simulink model "PID_Joint23_Simscape_Simulation"  (R2020b)
settings: Solver=ode2  StartTime=0.0  StopTime=20  FixedStep=Ts  RelTol=1e-3
model workspace (MAT data in the model file):
  Ts = 0.001
undefined symbols (not defined in the file): DiscIntNeverNeededParam, PositionControl, TorqueControl, X, Y, Z
libraries: sm_lib x112, nesl_utility x65, simulink x4, dspsrcs4 x2
(part 1 of 4)
settings Model: Creator=Jeason  LastModifiedBy=Administrator
settings DataIOCC: InspectSignalLogs=on  ReturnWorkspaceOutputs=off
settings DebuggingCC: ArithmeticOperatorsInVariantConditions=warning
settings SFSimCC: CustomCodeUndefinedFunction=UseInterfaceOnly

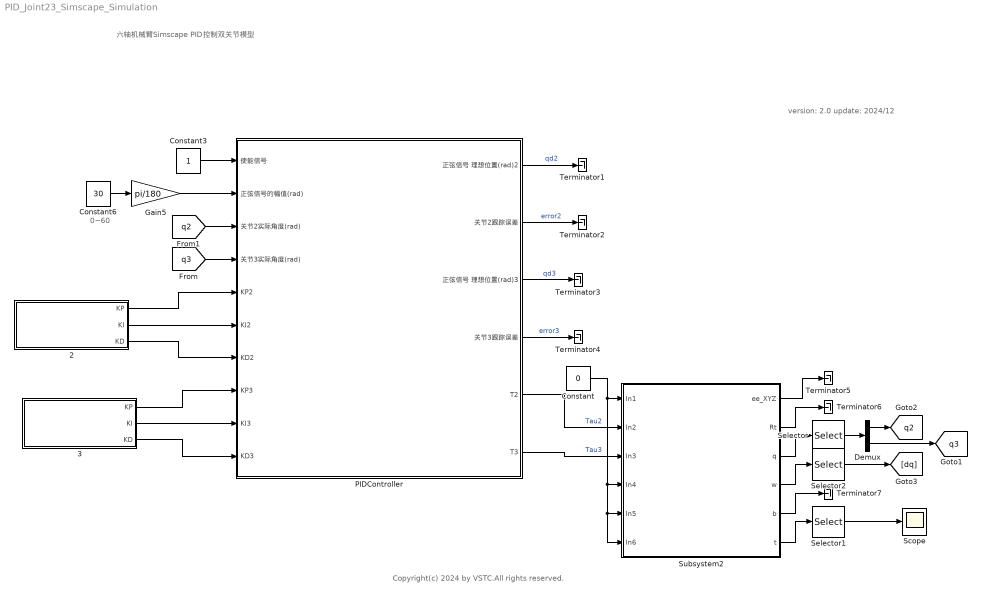
== system PID_Joint23_Simscape_Simulation ==
  note: 0~60
  note: 六轴机械臂Simscape PID控制双关节模型
  note: Copyright(c) 2024 by VSTC.All rights reserved.
  note: version: 2.0
      | update: 2024/12
  2 : Subsystem  mask{KP=300, KI=5, KD=10}
      mask DialogControl ParameterGroupVar Prompt: 参数
      mask Display: disp('PID parameters of Joint 2');
  3 : Subsystem  mask{KP=150, KI=5, KD=10}
      mask DialogControl ParameterGroupVar Prompt: 参数
      mask Display: disp('PID parameters of Joint 3');
  Constant : Constant  Value=0
  Constant3 : Constant
  Constant6 : Constant  Value=30
  Demux : Demux  Outputs=2
  Gain5 : Gain  Gain=pi/180
  PIDController : Subsystem  Priority=3  TreatAsAtomicUnit=on  RTWFcnName=AdaptiveAlgorithm
      settings: RTWSystemCode=Nonreusable function  RTWFcnNameOpts=User specified  RTWFileNameOpts=Use function name
  Scope : Scope
  Selector : Selector  InputPortWidth=6  IndexOptions=Index vector (dialog)  Indices=[2 3]  OutputSizes=1
  Selector1 : Selector  InputPortWidth=6  IndexOptions=Index vector (dialog)  Indices=3  OutputSizes=1
  Selector2 : Selector  InputPortWidth=6  IndexOptions=Index vector (dialog)  Indices=[2 3]  OutputSizes=1
  Subsystem2 : Subsystem  mask{VChoice1=PositionControl, VChoice2=TorqueControl, VChoice3=TorqueControl, VChoice4=PositionControl, VChoice5=PositionControl, VChoice6=PositionControl}
      mask prompts: VChoice1 "Select Joint1 Control Model"; VChoice2 "Select Joint2 Control Model"; VChoice3 "Select Joint3 Control Model"; VChoice4 "Select Joint4 Control Model"; VChoice5 "Select Joint5 Control Model"; VChoice6 "Select Joint6 Control Model"
      mask help: Model Choice
      mask TypeOptions VChoice1: Joint1/Variant Subsystem3/VChoice1
      mask TypeOptions VChoice2: Joint2/Variant Subsystem4/VChoice2
      mask TypeOptions VChoice3: Joint3/Variant Subsystem5/VChoice3
      mask TypeOptions VChoice4: Joint4/Variant Subsystem6/VChoice4
      mask TypeOptions VChoice5: Joint5/Variant Subsystem7/VChoice5
      mask TypeOptions VChoice6: Joint6/Variant Subsystem9/VChoice6
      mask Display:
      | % image('E:\SixRobotArm\Robot.png') ;
      | color('red');
      | disp('Six-DOF\n Collaborative Robot')
      | color('black');
      | choice1 = get_param(gcb,'VChoice1');
      | choice2 = get_param(gcb,'VChoice2');
      | choice3 = get_param(gcb,'VChoice3');
      | choice4 = get_param(gcb,'VChoice4');
      | choice5 = get_param(gcb,'VChoice5');
      | choice6 = get_param(gcb,'VChoice6');
      | if strcmp(choice1,'PositionControl') %TorqueControl
      |     port_label('input', 1, 'Theta1(rad)');
      | else
      |     port_label('input', 1, 'Torque1(N·m)');
      | end
      | if strcmp(choice2,'PositionControl') %TorqueControl
      |     port_label('input', 2, 'Theta2(rad)');
      | else
      |     port_label('input', 2, 'Torque2(N·m)');
      | end
      | if strcmp(choice3,'PositionControl') %TorqueControl
      |     port_label('input', 3, 'Theta3(rad)');
      | else
      |     port_label('input', 3, 'Torque3(N·m)');
      | end
      | if strcmp(choice4,'PositionControl') %TorqueControl
      |     port_label('input', 4, 'Theta4(rad)');
      | else
      |     port_label('input', 4, 'Torque4(N·m)');
      | end
      | if strcmp(choice5,'PositionControl') %TorqueControl
      |     port_label('input', 5, 'Theta5(rad)');
      | else
      |     port_label('input', 5, 'Torque5(N·m)');
      | end
      | if strcmp(choice6,'PositionControl') %TorqueControl
      |     port_label('input', 6, 'Theta6(rad)');
      | else
      |     port_label('input', 6, 'Torque6(N·m)');
      | end
      | 
      | port_label('output', 1, 'ee_XYZ(mm)');
      | port_label('output', 2, 'Rotation matrix');
      | port_label('output', 3, 'Angle(rad)');
      | port_label('output', 4, 'Vel(rad/s)');
      | port_label('output', 5, 'Acc(rad/s^2)');
      | port_label('output', 6, 'Torque(N·m)');
  Terminator{1..7} (7 alike) : Terminator
  tag scope: q2=global, q3=global
  wires:
  Gain5/1 -> PIDController/2(正弦信号的幅值(rad))
  Constant6/1 -> Gain5/1
  Constant3/1 -> PIDController/1(使能信号)
  [q3] -> PIDController/4(关节3实际角度(rad))
  [q2] -> PIDController/3(关节2实际角度(rad))
  2/1(KP) -> PIDController/5(KP2)
  2/2(KI) -> PIDController/6(KI2)
  2/3(KD) -> PIDController/7(KD2)
  3/1(KP) -> PIDController/8(KP3)
  3/2(KI) -> PIDController/9(KI3)
  3/3(KD) -> PIDController/10(KD3)
  PIDController/1(正弦信号 理想位置(rad)2) -> Terminator1/1  "qd2"
  PIDController/2(关节2跟踪误差) -> Terminator2/1  "error2"
  PIDController/3(正弦信号 理想位置(rad)3) -> Terminator3/1  "qd3"
  PIDController/4(关节3跟踪误差) -> Terminator4/1  "error3"
  Selector/1 -> Demux/1
  Selector1/1 -> Scope/1
  Selector2/1 -> [dq]
  Constant/1 -> Subsystem2/1(In1), Subsystem2/6(In6), Subsystem2/5(In5), Subsystem2/4(In4)
  Demux/1 -> [q2]
  Demux/2 -> [q3]
  Subsystem2/1(ee_XYZ) -> Terminator5/1
  Subsystem2/2(Rt) -> Terminator6/1
  Subsystem2/3(q) -> Selector/1
  Subsystem2/4(w) -> Selector2/1
  Subsystem2/5(b) -> Terminator7/1
  Subsystem2/6(t) -> Selector1/1
  PIDController/6(T3) -> Subsystem2/3(In3)  "Tau3"
  PIDController/5(T2) -> Subsystem2/2(In2)  "Tau2"

== system PID_Joint23_Simscape_Simulation/2 ==
  Constant : Constant  Value=KP
  Constant1 : Constant  Value=KI
  Constant2 : Constant  Value=KD
  KP : Outport
  KI : Outport  Port=2
  KD : Outport  Port=3
  wires:
  Constant/1 -> KP/1
  Constant1/1 -> KI/1
  Constant2/1 -> KD/1

== system PID_Joint23_Simscape_Simulation/3 ==
  Constant : Constant  Value=KP
  Constant1 : Constant  Value=KI
  Constant2 : Constant  Value=KD
  KP : Outport
  KI : Outport  Port=2
  KD : Outport  Port=3
  wires:
  Constant1/1 -> KI/1
  Constant2/1 -> KD/1
  Constant/1 -> KP/1

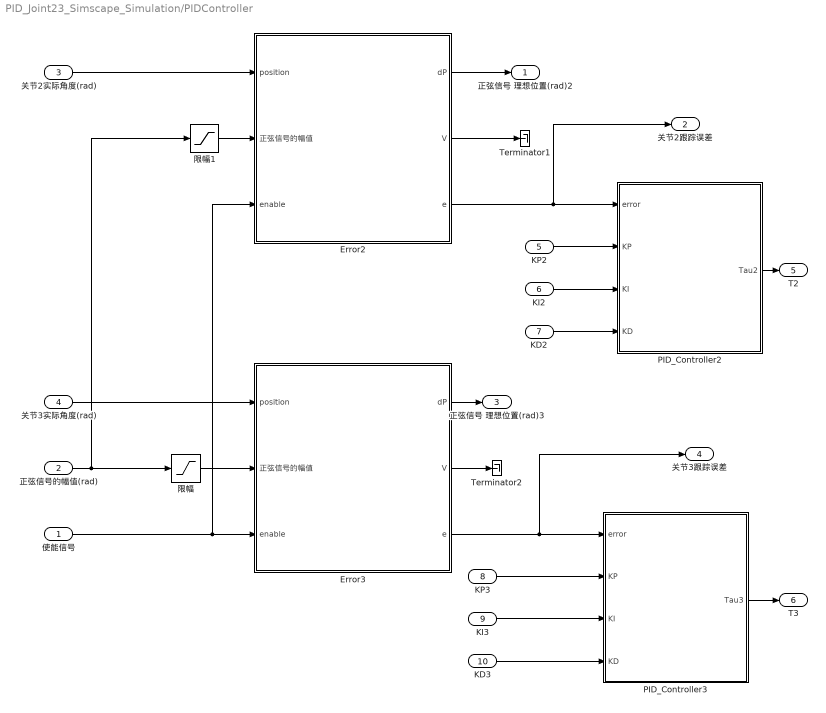
== system PID_Joint23_Simscape_Simulation/PIDController ==
  使能信号 : Inport
  正弦信号的幅值(rad) : Inport  Port=2
  关节2实际角度(rad) : Inport  Port=3
  关节3实际角度(rad) : Inport  Port=4
  KP2 : Inport  Port=5
  KI2 : Inport  Port=6
  KD2 : Inport  Port=7
  KP3 : Inport  Port=8
  KI3 : Inport  Port=9
  KD3 : Inport  Port=10
  Error2 : Subsystem  Priority=1  TreatAsAtomicUnit=on
      settings: RTWSystemCode=Nonreusable function  RTWFcnNameOpts=Use subsystem name  FunctionInterfaceSpec=Allow arguments (Optimized)
  Error3 : Subsystem  Priority=1  TreatAsAtomicUnit=on
      settings: RTWSystemCode=Nonreusable function  RTWFcnNameOpts=Use subsystem name  FunctionInterfaceSpec=Allow arguments (Optimized)
  PID_Controller2 : Subsystem  TreatAsAtomicUnit=on
      settings: RTWSystemCode=Nonreusable function
  PID_Controller3 : Subsystem  TreatAsAtomicUnit=on
      settings: RTWSystemCode=Nonreusable function
  Terminator1 : Terminator
  Terminator2 : Terminator
  限幅 : Saturate  UpperLimit=pi/3  LowerLimit=0
  限幅1 : Saturate  UpperLimit=pi/3  LowerLimit=0
  正弦信号 理想位置(rad)2 : Outport  VectorParamsAs1DForOutWhenUnconnected=off
  关节2跟踪误差 : Outport  Port=2  VectorParamsAs1DForOutWhenUnconnected=off
  正弦信号 理想位置(rad)3 : Outport  Port=3  VectorParamsAs1DForOutWhenUnconnected=off
  关节3跟踪误差 : Outport  Port=4  VectorParamsAs1DForOutWhenUnconnected=off
  T2 : Outport  Port=5  VectorParamsAs1DForOutWhenUnconnected=off
  T3 : Outport  Port=6  VectorParamsAs1DForOutWhenUnconnected=off
  wires:
  关节3实际角度(rad)/1 -> Error3/1(position)
  限幅/1 -> Error3/2(正弦信号的幅值)
  使能信号/1 -> Error2/3(enable), Error3/3(enable)
  Error3/3(e) -> 关节3跟踪误差/1, PID_Controller3/1(error)
  KP3/1 -> PID_Controller3/2(KP)
  KI3/1 -> PID_Controller3/3(KI)
  KD3/1 -> PID_Controller3/4(KD)
  Error3/1(dP) -> 正弦信号 理想位置(rad)3/1
  Error3/2(V) -> Terminator2/1
  Error2/3(e) -> 关节2跟踪误差/1, PID_Controller2/1(error)
  Error2/1(dP) -> 正弦信号 理想位置(rad)2/1
  Error2/2(V) -> Terminator1/1
  关节2实际角度(rad)/1 -> Error2/1(position)
  限幅1/1 -> Error2/2(正弦信号的幅值)
  KD2/1 -> PID_Controller2/4(KD)
  KI2/1 -> PID_Controller2/3(KI)
  KP2/1 -> PID_Controller2/2(KP)
  PID_Controller3/1(Tau3) -> T3/1
  PID_Controller2/1(Tau2) -> T2/1
  正弦信号的幅值(rad)/1 -> 限幅/1, 限幅1/1

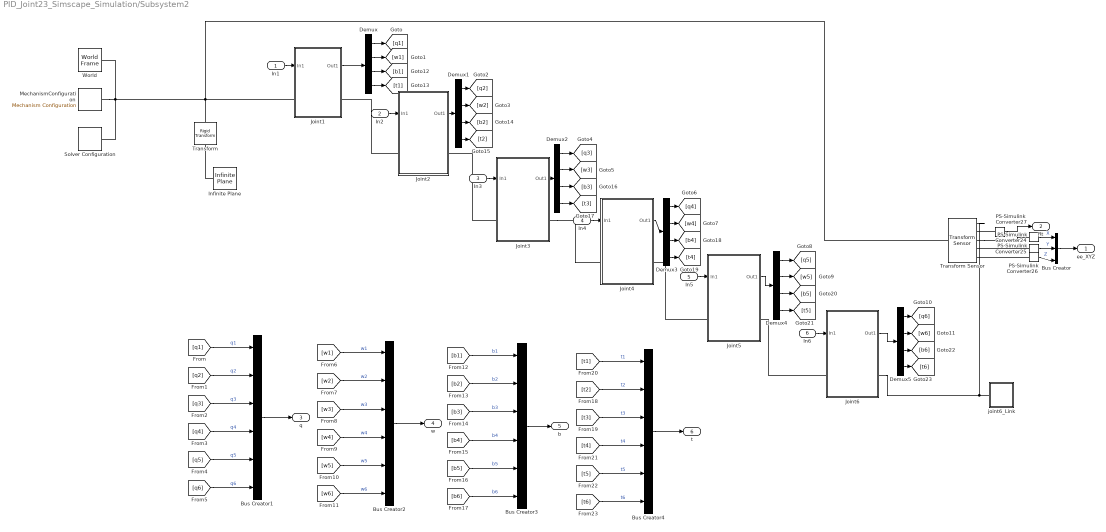
== system PID_Joint23_Simscape_Simulation/Subsystem2 ==
  In1 : Inport
  In2 : Inport  Port=2
  In3 : Inport  Port=3
  In4 : Inport  Port=4
  In5 : Inport  Port=5
  In6 : Inport  Port=6
  Bus Creator : BusCreator  Inputs=3
  Bus Creator{1..4} (4 alike) : BusCreator  Inputs=6
  Demux{,1..5} (6 alike) : Demux
  Infinite Plane : sm_lib/Curves and Surfaces/Infinite Plane  GraphicType=Rectangle  GraphicPlaneWidth=1  GraphicPlaneWidthUnits=m  GraphicPlaneHeight=1  GraphicPlaneHeightUnits=m  GraphicVisPropType=SimpleVisualProperties  GraphicDiffuseColor=[0.5 0.5 0.5]  GraphicOpacity=1  GraphicSpecularColor=[0.5 0.5 0.5 1.0]  GraphicAmbientColor=[0.15 0.15 0.15 1.0]  GraphicEmissiveColor=[0.0 0.0 0.0 1.0]  GraphicShininess=75
  Joint1 : Subsystem
  Joint2 : Subsystem
  Joint3 : Subsystem
  Joint4 : Subsystem
  Joint5 : Subsystem
  Joint6 : Subsystem
  MechanismConfiguration : sm_lib/Utilities/Mechanism Configuration  UniformGravity=Constant  GravityVector=[0 0 -9.80665]  GravityVectorUnits=m/s^2  GravityUnits=m/s^2  LinearizationDelta=0.001  JointModeTransitionNonlinearIterations=2
  PS-Simulink Converter{24..27} (4 alike) : nesl_utility/PS-Simulink Converter  PhysicalDomain=network_engine_domain  SubClassName=ps_output  LeftPortType=input  RightPortType=output  PseudoPeriodic=off  Frequencies=[]  Unit=mm  AffineConversion=off
      settings: SourceProductBaseCode=PW,SS
  Solver Configuration : nesl_utility/Solver Configuration  PhysicalDomain=network_engine_domain  SubClassName=solver  LeftPortType=input  RightPortType=generic  Tones=[]  Harmonics=[]  SimulateNoise=off  Profile=off  UseLocalSampling=off  EnableSwitchedLinearOptims=on  FrequencyDomain=off  UseCCode=off  RelTol=0.001  AbsTol=1e-06  MinStep=1e-09  ToWorkspace=off  RevertToSquareIcSolve=off  NumHomotopyIterations=100  PhasorMode=off  PhasorModeNumHarmonics=1  DoDC=off  ResidualTolerance=1e-09  UseLocalSolver=off  LocalSolverChoice=NE_BACKWARD_EULER_ADVANCER  LocalSolverSampleTime=0.001  DoFixedCost=off  MaxNonlinIter=3  MaxModeIter=2  ComputeImpulses=off  ImpulseIterations=2  LinearAlgebra=auto  EquationFormulation=NE_TIME_EF  DelaysMemoryBudget=1024  AutomaticFiltering=on  FilteringTimeConstant=0.001  PartitionStorageMethod=AS_NEEDED  PartitionMemoryBudget=1024  PartitionMethod=ROBUST
  Transform : sm_lib/Frames and Transforms/Rigid Transform  TranslationMethod=Cartesian  TranslationStandardOffset=0  TranslationLengthUnit=m  TranslationStandardAxis=+Z  TranslationCartesianOffset=[0, 0, 0]  TranslationROffset=0  TranslationROffsetUnits=m  TranslationZOffset=0  TranslationZOffsetUnits=m  TranslationThetaOffset=0  TranslationThetaOffsetUnits=deg  RotationMethod=RotationSequence  RotationAngleUnits=deg  RotationStandardAxis=+Z  RotationAngle=0.0  RotationArbitraryAxis=[0 0 1]  FollAlignAxisA=+X  BaseAlignAxisA=+Y  FollAlignAxisB=+Y  BaseAlignAxisB=+Z  RotationSequenceAxes=BaseAxes  RotationSequence=XYZ  RotationSequenceAngles=[0, 0, 0]  RotationSequenceAnglesUnits=rad  RotationMatrix=[1 0 0; 0 1 0; 0 0 1]
  Transform Sensor : sm_lib/Frames and Transforms/Transform Sensor  MeasurementFrame=Base  SenseAngle=off  SenseAxis=off  SenseAngle1=off  SenseAngle2=off  SenseAngle3=off  SenseQ=off  SenseR=on  SenseOmegaX=off  SenseOmegaY=off  SenseOmegaZ=off  SenseOmega1=off  SenseOmega2=off  SenseOmega3=off  SenseQDot=off  SenseRDot=off  SenseAlphaX=off  SenseAlphaY=off  SenseAlphaZ=off  SenseAlpha1=off  SenseAlpha2=off  SenseAlpha3=off  SenseQDDot=off  SenseRDDot=off  SenseX=on  SenseY=on  SenseZ=on  SenseRad=off  SenseAzim=off  SenseDist=off  SenseInc=off  SenseXDot=off  SenseYDot=off  SenseZDot=off  SenseRadDot=off  SenseAzimDot=off  SenseDistDot=off  SenseIncDot=off  SenseXDDot=off  SenseYDDot=off  SenseZDDot=off  SenseRadDDot=off  SenseAzimDDot=off  SenseDistDDot=off  SenseIncDDot=off
  World : sm_lib/Frames and Transforms/World Frame
  joint6_Link : Subsystem
  ee_XYZ : Outport
  Rt : Outport  Port=2
  q : Outport  Port=3
  w : Outport  Port=4
  b : Outport  Port=5
  t : Outport  Port=6
  wires:
  Demux4/4 -> [t5]
  PS-Simulink Converter25/1 -> Bus Creator/2  "Y"
  Joint3/1(Out1) -> Demux2/1
  Joint6/1(Out1) -> Demux5/1
  Demux3/4 -> [t4]
  PS-Simulink Converter26/1 -> Bus Creator/3  "Z"
  [q6] -> Bus Creator1/6  "q6"
  [b1] -> Bus Creator3/1  "b1"
  Joint4/1(Out1) -> Demux3/1
  [q1] -> Bus Creator1/1  "q1"
  Demux/3 -> [b1]
  Demux4/3 -> [b5]
  [t2] -> Bus Creator4/2  "t2"
  Bus Creator2/1 -> w/1
  Demux1/4 -> [t2]
  Joint1/1(Out1) -> Demux/1
  [w4] -> Bus Creator2/4  "w4"
  Demux4/2 -> [w5]
  Demux2/4 -> [t3]
  [q3] -> Bus Creator1/3  "q3"
  Demux/1 -> [q1]
  Demux1/3 -> [b2]
  [b5] -> Bus Creator3/5  "b5"
  Demux2/3 -> [b3]
  Demux2/1 -> [q3]
  [w3] -> Bus Creator2/3  "w3"
  [b2] -> Bus Creator3/2  "b2"
  [t5] -> Bus Creator4/5  "t5"
  [q4] -> Bus Creator1/4  "q4"
  Demux/2 -> [w1]
  Demux3/3 -> [b4]
  Bus Creator/1 -> ee_XYZ/1
  Demux5/3 -> [b6]
  [t6] -> Bus Creator4/6  "t6"
  Demux/4 -> [t1]
  Bus Creator1/1 -> q/1
  Demux5/1 -> [q6]
  [w6] -> Bus Creator2/6  "w6"
  PS-Simulink Converter27/1 -> Rt/1
  [w5] -> Bus Creator2/5  "w5"
  [q2] -> Bus Creator1/2  "q2"
  In4/1 -> Joint4/1(In1)
  In6/1 -> Joint6/1(In1)
  In5/1 -> Joint5/1(In1)
  [b3] -> Bus Creator3/3  "b3"
  Demux1/1 -> [q2]
  Demux3/1 -> [q4]
  In3/1 -> Joint3/1(In1)
  [q5] -> Bus Creator1/5  "q5"
  [w1] -> Bus Creator2/1  "w1"
  Bus Creator3/1 -> b/1
  PS-Simulink Converter24/1 -> Bus Creator/1  "X"
  [b6] -> Bus Creator3/6  "b6"
  [t3] -> Bus Creator4/3  "t3"
  [t1] -> Bus Creator4/1  "t1"
  [w2] -> Bus Creator2/2  "w2"
  Joint5/1(Out1) -> Demux4/1
  [t4] -> Bus Creator4/4  "t4"
  Demux1/2 -> [w2]
  Demux4/1 -> [q5]
  Demux2/2 -> [w3]
  In2/1 -> Joint2/1(In1)
  In1/1 -> Joint1/1(In1)
  Demux3/2 -> [w4]
  Joint2/1(Out1) -> Demux1/1
  Bus Creator4/1 -> t/1
  Demux5/2 -> [w6]
  [b4] -> Bus Creator3/4  "b4"
  Demux5/4 -> [t6]
  connections:
  Joint1/LConn1 -- World/RConn1 -- MechanismConfiguration/RConn1 -- Solver Configuration/RConn1 -- Transform/LConn1 -- Transform Sensor/LConn1
  Infinite Plane/LConn1 -- Transform/RConn1
  Transform Sensor/RConn3 -- PS-Simulink Converter24/LConn1
  PS-Simulink Converter27/LConn1 -- Transform Sensor/RConn2
  Joint3/RConn1 -- Joint4/LConn1
  Joint6/LConn1 -- Joint5/RConn1
  PS-Simulink Converter26/LConn1 -- Transform Sensor/RConn5
  PS-Simulink Converter25/LConn1 -- Transform Sensor/RConn4
  Joint2/LConn1 -- Joint1/RConn1
  Joint5/LConn1 -- Joint4/RConn1
  Joint3/LConn1 -- Joint2/RConn1
  Joint6/RConn1 -- Transform Sensor/RConn1 -- joint6_Link/LConn1

== system PID_Joint23_Simscape_Simulation/PIDController/Error2 ==
  note: $e_1(t)=\theta(t)-\theta_d(t)$
  note: $\dot\theta_d(t)$
  position : Inport
  正弦信号的幅值 : Inport  Port=2
  enable : Inport  Port=3
  Discrete Derivative : simulink/Discrete/Discrete Derivative  gainval=1.0  ICPrevScaledInput=0.0  OutMin=[]  OutMax=[]  OutDataType=fixdt(1, 16)  OutScaling=2^-10  DoSatur=off
  Subsystem : Subsystem
      settings: RTWSystemCode=Nonreusable function
  dP : Outport  VectorParamsAs1DForOutWhenUnconnected=off
  V : Outport  Port=2  VectorParamsAs1DForOutWhenUnconnected=off
  e : Outport  Port=3  VectorParamsAs1DForOutWhenUnconnected=off
  wires:
  position/1 -> Subsystem/1(position)
  Discrete Derivative/1 -> V/1
  enable/1 -> Subsystem/Enable
  Subsystem/2(理想位置) -> dP/1, Discrete Derivative/1
  Subsystem/1(e1) -> e/1
  正弦信号的幅值/1 -> Subsystem/2(Amplitude)

== system PID_Joint23_Simscape_Simulation/PIDController/Error3 ==
  note: $e_1(t)=\theta(t)-\theta_d(t)$
  note: $\dot\theta_d(t)$
  position : Inport
  正弦信号的幅值 : Inport  Port=2
  enable : Inport  Port=3
  Discrete Derivative : simulink/Discrete/Discrete Derivative  gainval=1.0  ICPrevScaledInput=0.0  OutMin=[]  OutMax=[]  OutDataType=fixdt(1, 16)  OutScaling=2^-10  DoSatur=off
  Subsystem : Subsystem
      settings: RTWSystemCode=Nonreusable function
  dP : Outport  VectorParamsAs1DForOutWhenUnconnected=off
  V : Outport  Port=2  VectorParamsAs1DForOutWhenUnconnected=off
  e : Outport  Port=3  VectorParamsAs1DForOutWhenUnconnected=off
  wires:
  position/1 -> Subsystem/1(position)
  Discrete Derivative/1 -> V/1
  enable/1 -> Subsystem/Enable
  Subsystem/2(理想位置) -> dP/1, Discrete Derivative/1
  Subsystem/1(e1) -> e/1
  正弦信号的幅值/1 -> Subsystem/2(Amplitude)

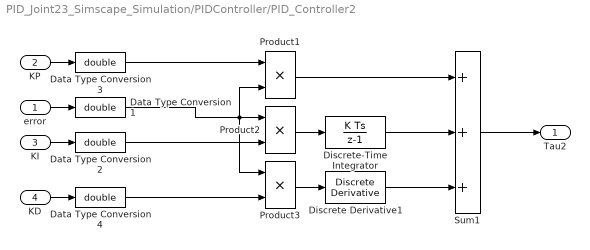
== system PID_Joint23_Simscape_Simulation/PIDController/PID_Controller2 ==
  error : Inport
  KP : Inport  Port=2
  KI : Inport  Port=3
  KD : Inport  Port=4
  Data Type Conversion{1..4} (4 alike) : DataTypeConversion  OutDataTypeStr=double
  Discrete Derivative1 : simulink/Discrete/Discrete Derivative  gainval=1.0  ICPrevScaledInput=0.0  OutMin=[]  OutMax=[]  OutDataType=fixdt(1, 16)  OutScaling=2^-10  DoSatur=off
  Discrete-Time Integrator : DiscreteIntegrator  SampleTime=-1  ICPrevOutput=DiscIntNeverNeededParam  ICPrevScaledInput=DiscIntNeverNeededParam
  Product1 : Product
  Product2 : Product
  Product3 : Product
  Sum1 : Sum  Inputs=+++
  Tau2 : Outport  VectorParamsAs1DForOutWhenUnconnected=off
  wires:
  Product2/1 -> Discrete-Time Integrator/1
  error/1 -> Data Type Conversion1/1
  Product3/1 -> Discrete Derivative1/1
  KP/1 -> Data Type Conversion3/1
  Sum1/1 -> Tau2/1
  Discrete Derivative1/1 -> Sum1/3
  Product1/1 -> Sum1/1
  Discrete-Time Integrator/1 -> Sum1/2
  KI/1 -> Data Type Conversion2/1
  KD/1 -> Data Type Conversion4/1
  Data Type Conversion3/1 -> Product1/1
  Data Type Conversion4/1 -> Product3/2
  Data Type Conversion2/1 -> Product2/2
  Data Type Conversion1/1 -> Product3/1, Product1/2, Product2/1

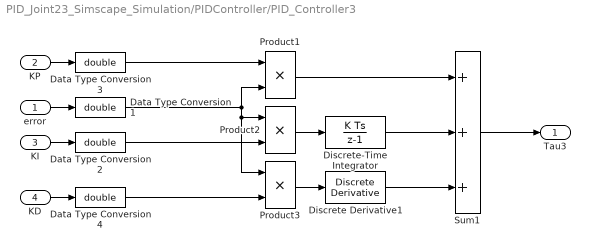
== system PID_Joint23_Simscape_Simulation/PIDController/PID_Controller3 ==
  error : Inport
  KP : Inport  Port=2
  KI : Inport  Port=3
  KD : Inport  Port=4
  Data Type Conversion{1..4} (4 alike) : DataTypeConversion  OutDataTypeStr=double
  Discrete Derivative1 : simulink/Discrete/Discrete Derivative  gainval=1.0  ICPrevScaledInput=0.0  OutMin=[]  OutMax=[]  OutDataType=fixdt(1, 16)  OutScaling=2^-10  DoSatur=off
  Discrete-Time Integrator : DiscreteIntegrator  SampleTime=-1  ICPrevOutput=DiscIntNeverNeededParam  ICPrevScaledInput=DiscIntNeverNeededParam
  Product1 : Product
  Product2 : Product
  Product3 : Product
  Sum1 : Sum  Inputs=+++
  Tau3 : Outport  VectorParamsAs1DForOutWhenUnconnected=off
  wires:
  Product2/1 -> Discrete-Time Integrator/1
  error/1 -> Data Type Conversion1/1
  Product3/1 -> Discrete Derivative1/1
  KP/1 -> Data Type Conversion3/1
  Sum1/1 -> Tau3/1
  Discrete Derivative1/1 -> Sum1/3
  Product1/1 -> Sum1/1
  Discrete-Time Integrator/1 -> Sum1/2
  KI/1 -> Data Type Conversion2/1
  KD/1 -> Data Type Conversion4/1
  Data Type Conversion1/1 -> Product1/2, Product3/1, Product2/1
  Data Type Conversion3/1 -> Product1/1
  Data Type Conversion4/1 -> Product3/2
  Data Type Conversion2/1 -> Product2/2

== system PID_Joint23_Simscape_Simulation/Subsystem2/Joint1 ==
  In1 : Inport
  Variant Subsystem3 : Subsystem  Variant=on  VariantControlMode=label  LabelModeActiveChoice=PositionControl  mask{VChoice1=PositionControl, LowerBound=-180, UpperBound=180}
      mask prompts: VChoice1 "Select Control Model"; LowerBound "LowerBound(deg"; UpperBound "UpperBound(deg)"
      mask help: Joint1 Control Model
      mask init:
      | choice = get_param(gcb,'VChoice1');
      | vssBlk = gcb;
      | oldVariant = get_param(gcb,'LabelModeActiveChoice');
      | if strcmp(choice,'PositionControl')
      |     
      |     set_param(vssBlk, 'LabelModeActiveChoice', 'PositionControl');
      | elseif strcmp(choice,'TorqueControl')
      |     
      |     set_param(vssBlk, 'LabelModeActiveChoice', 'TorqueControl');
      | end
      mask TypeOptions VChoice1: PositionControl | TorqueControl
  base_link : Subsystem
  BaseConn : PMIOPort  Side=Left
  Conn1 : PMIOPort  Port=2  Side=Right
  Out1 : Outport
  wires:
  Variant Subsystem3/1(Out1) -> Out1/1
  In1/1 -> Variant Subsystem3/1(In1)
  connections:
  Variant Subsystem3/LConn1 -- base_link/RConn1
  Variant Subsystem3/RConn1 -- Conn1/RConn1
  BaseConn/RConn1 -- base_link/LConn1

== system PID_Joint23_Simscape_Simulation/Subsystem2/Joint2 ==
  In1 : Inport
  Variant Subsystem4 : Subsystem  Variant=on  VariantControlMode=label  LabelModeActiveChoice=TorqueControl  mask{VChoice2=TorqueControl, LowerBound=-180, UpperBound=180}
      mask prompts: VChoice2 "Select Control Model"; LowerBound "LowerBound(deg"; UpperBound "UpperBound(deg)"
      mask help: Joint2 Control Model
      mask init:
      | choice = get_param(gcb,'VChoice2');
      | vssBlk = gcb;
      | oldVariant = get_param(gcb,'LabelModeActiveChoice');
      | if strcmp(choice,'PositionControl')
      |     
      |     set_param(vssBlk, 'LabelModeActiveChoice', 'PositionControl');
      | elseif strcmp(choice,'TorqueControl')
      |     
      |     set_param(vssBlk, 'LabelModeActiveChoice', 'TorqueControl');
      | end
      mask TypeOptions VChoice2: PositionControl | TorqueControl
  joint1_Link : Subsystem
  joint1_x1 : sm_lib/Joints/Weld Joint  JointMode=Normal  SenseConstraintForce=off  SenseConstraintForceX=off  SenseConstraintForceY=off  SenseConstraintForceZ=off  SenseConstraintTorque=off  SenseConstraintTorqueX=off  SenseConstraintTorqueY=off  SenseConstraintTorqueZ=off  SenseTotalForce=off  SenseTotalForceX=off  SenseTotalForceY=off  SenseTotalForceZ=off  SenseTotalTorque=off  SenseTotalTorqueX=off  SenseTotalTorqueY=off  SenseTotalTorqueZ=off  CompositeWrenchDir=FollowerOnBase  CompositeWrenchFrame=BaseFrame
  joint1_x1_Link : Subsystem
  joint1_x2 : sm_lib/Joints/Weld Joint  JointMode=Normal  SenseConstraintForce=off  SenseConstraintForceX=off  SenseConstraintForceY=off  SenseConstraintForceZ=off  SenseConstraintTorque=off  SenseConstraintTorqueX=off  SenseConstraintTorqueY=off  SenseConstraintTorqueZ=off  SenseTotalForce=off  SenseTotalForceX=off  SenseTotalForceY=off  SenseTotalForceZ=off  SenseTotalTorque=off  SenseTotalTorqueX=off  SenseTotalTorqueY=off  SenseTotalTorqueZ=off  CompositeWrenchDir=FollowerOnBase  CompositeWrenchFrame=BaseFrame
  joint1_x2_Link : Subsystem
  Conn1 : PMIOPort  Side=Left
  Conn2 : PMIOPort  Port=2  Side=Right
  Out1 : Outport
  wires:
  Variant Subsystem4/1(Out1) -> Out1/1
  In1/1 -> Variant Subsystem4/1(In1)
  connections:
  Conn1/RConn1 -- joint1_Link/LConn1
  Variant Subsystem4/RConn1 -- Conn2/RConn1
  joint1_x2/RConn1 -- joint1_x2_Link/LConn1
  joint1_Link/RConn2 -- joint1_x2/LConn1
  joint1_Link/RConn3 -- joint1_x1/LConn1
  joint1_x1/RConn1 -- joint1_x1_Link/LConn1
  joint1_Link/RConn1 -- Variant Subsystem4/LConn1

== system PID_Joint23_Simscape_Simulation/Subsystem2/Joint3 ==
  In1 : Inport
  Variant Subsystem5 : Subsystem  Variant=on  VariantControlMode=label  LabelModeActiveChoice=TorqueControl  mask{VChoice3=TorqueControl, LowerBound=-180, UpperBound=180}
      mask prompts: VChoice3 "Select Control Model"; LowerBound "LowerBound(deg"; UpperBound "UpperBound(deg)"
      mask help: Joint3 Control Model
      mask init:
      | choice = get_param(gcb,'VChoice3');
      | vssBlk = gcb;
      | oldVariant = get_param(gcb,'LabelModeActiveChoice');
      | if strcmp(choice,'PositionControl')
      |     
      |     set_param(vssBlk, 'LabelModeActiveChoice', 'PositionControl');
      | elseif strcmp(choice,'TorqueControl')
      |     
      |     set_param(vssBlk, 'LabelModeActiveChoice', 'TorqueControl');
      | end
      mask TypeOptions VChoice3: PositionControl | TorqueControl
  joint2_Link : Subsystem
  joint2_x1 : sm_lib/Joints/Weld Joint  JointMode=Normal  SenseConstraintForce=off  SenseConstraintForceX=off  SenseConstraintForceY=off  SenseConstraintForceZ=off  SenseConstraintTorque=off  SenseConstraintTorqueX=off  SenseConstraintTorqueY=off  SenseConstraintTorqueZ=off  SenseTotalForce=off  SenseTotalForceX=off  SenseTotalForceY=off  SenseTotalForceZ=off  SenseTotalTorque=off  SenseTotalTorqueX=off  SenseTotalTorqueY=off  SenseTotalTorqueZ=off  CompositeWrenchDir=FollowerOnBase  CompositeWrenchFrame=BaseFrame
  joint2_x1_Link : Subsystem
  Conn2 : PMIOPort  Side=Left
  Conn3 : PMIOPort  Port=2  Side=Right
  Out1 : Outport
  wires:
  In1/1 -> Variant Subsystem5/1(In1)
  Variant Subsystem5/1(Out1) -> Out1/1
  connections:
  Variant Subsystem5/LConn1 -- joint2_Link/RConn1
  Conn2/RConn1 -- joint2_Link/LConn1
  Variant Subsystem5/RConn1 -- Conn3/RConn1
  joint2_x1/RConn1 -- joint2_x1_Link/LConn1
  joint2_Link/RConn2 -- joint2_x1/LConn1

== system PID_Joint23_Simscape_Simulation/Subsystem2/Joint4 ==
  In1 : Inport
  Variant Subsystem6 : Subsystem  Variant=on  VariantControlMode=label  LabelModeActiveChoice=PositionControl  mask{VChoice4=PositionControl, LowerBound=-180, UpperBound=180}
      mask prompts: VChoice4 "Select Control Model"; LowerBound "LowerBound(deg"; UpperBound "UpperBound(deg)"
      mask help: Joint4 Control Model
      mask init:
      | choice = get_param(gcb,'VChoice4');
      | vssBlk = gcb;
      | oldVariant = get_param(gcb,'LabelModeActiveChoice');
      | if strcmp(choice,'PositionControl')
      |     
      |     set_param(vssBlk, 'LabelModeActiveChoice', 'PositionControl');
      | elseif strcmp(choice,'TorqueControl')
      |     
      |     set_param(vssBlk, 'LabelModeActiveChoice', 'TorqueControl');
      | end
      mask TypeOptions VChoice4: PositionControl | TorqueControl
  joint3_Link : Subsystem
  joint3_x1 : sm_lib/Joints/Weld Joint  JointMode=Normal  SenseConstraintForce=off  SenseConstraintForceX=off  SenseConstraintForceY=off  SenseConstraintForceZ=off  SenseConstraintTorque=off  SenseConstraintTorqueX=off  SenseConstraintTorqueY=off  SenseConstraintTorqueZ=off  SenseTotalForce=off  SenseTotalForceX=off  SenseTotalForceY=off  SenseTotalForceZ=off  SenseTotalTorque=off  SenseTotalTorqueX=off  SenseTotalTorqueY=off  SenseTotalTorqueZ=off  CompositeWrenchDir=FollowerOnBase  CompositeWrenchFrame=BaseFrame
  joint3_x1_Link : Subsystem
  Conn3 : PMIOPort  Side=Left
  Conn4 : PMIOPort  Port=2  Side=Right
  Out1 : Outport
  wires:
  In1/1 -> Variant Subsystem6/1(In1)
  Variant Subsystem6/1(Out1) -> Out1/1
  connections:
  Variant Subsystem6/LConn1 -- joint3_Link/RConn1
  joint3_Link/LConn1 -- Conn3/RConn1
  Variant Subsystem6/RConn1 -- Conn4/RConn1
  joint3_Link/RConn2 -- joint3_x1/LConn1
  joint3_x1/RConn1 -- joint3_x1_Link/LConn1

== system PID_Joint23_Simscape_Simulation/Subsystem2/Joint5 ==
  In1 : Inport
  Variant Subsystem7 : Subsystem  Variant=on  VariantControlMode=label  LabelModeActiveChoice=PositionControl  mask{VChoice5=PositionControl, LowerBound=-180, UpperBound=180}
      mask prompts: VChoice5 "Select Control Model"; LowerBound "LowerBound(deg"; UpperBound "UpperBound(deg)"
      mask help: Joint5 Control Model
      mask init:
      | choice = get_param(gcb,'VChoice5');
      | vssBlk = gcb;
      | oldVariant = get_param(gcb,'LabelModeActiveChoice');
      | if strcmp(choice,'PositionControl')
      |     
      |     set_param(vssBlk, 'LabelModeActiveChoice', 'PositionControl');
      | elseif strcmp(choice,'TorqueControl')
      |     
      |     set_param(vssBlk, 'LabelModeActiveChoice', 'TorqueControl');
      | end
      mask TypeOptions VChoice5: PositionControl | TorqueControl
  joint4_Link : Subsystem
  joint4_x1 : sm_lib/Joints/Weld Joint  JointMode=Normal  SenseConstraintForce=off  SenseConstraintForceX=off  SenseConstraintForceY=off  SenseConstraintForceZ=off  SenseConstraintTorque=off  SenseConstraintTorqueX=off  SenseConstraintTorqueY=off  SenseConstraintTorqueZ=off  SenseTotalForce=off  SenseTotalForceX=off  SenseTotalForceY=off  SenseTotalForceZ=off  SenseTotalTorque=off  SenseTotalTorqueX=off  SenseTotalTorqueY=off  SenseTotalTorqueZ=off  CompositeWrenchDir=FollowerOnBase  CompositeWrenchFrame=BaseFrame
  joint4_x1_Link : Subsystem
  Conn4 : PMIOPort  Side=Left
  Conn5 : PMIOPort  Port=2  Side=Right
  Out1 : Outport
  wires:
  In1/1 -> Variant Subsystem7/1(In1)
  Variant Subsystem7/1(Out1) -> Out1/1
  connections:
  joint4_Link/LConn1 -- Conn4/RConn1
  Conn5/RConn1 -- Variant Subsystem7/RConn1
  joint4_Link/RConn2 -- joint4_x1/LConn1
  joint4_x1/RConn1 -- joint4_x1_Link/LConn1
  joint4_Link/RConn1 -- Variant Subsystem7/LConn1

== system PID_Joint23_Simscape_Simulation/Subsystem2/Joint6 ==
  In1 : Inport
  Variant Subsystem9 : Subsystem  Variant=on  VariantControlMode=label  LabelModeActiveChoice=PositionControl  mask{VChoice6=PositionControl, LowerBound=-180, UpperBound=180}
      mask prompts: VChoice6 "Select Control Model"; LowerBound "LowerBound(deg"; UpperBound "UpperBound(deg)"
      mask help: Joint6 Control Model
      mask init:
      | choice = get_param(gcb,'VChoice6');
      | vssBlk = gcb;
      | oldVariant = get_param(gcb,'LabelModeActiveChoice');
      | if strcmp(choice,'PositionControl')
      |     
      |     set_param(vssBlk, 'LabelModeActiveChoice', 'PositionControl');
      | elseif strcmp(choice,'TorqueControl')
      |     
      |     set_param(vssBlk, 'LabelModeActiveChoice', 'TorqueControl');
      | end
      mask TypeOptions VChoice6: PositionControl | TorqueControl
  joint5_Link : Subsystem
  joint5_x1 : sm_lib/Joints/Weld Joint  JointMode=Normal  SenseConstraintForce=off  SenseConstraintForceX=off  SenseConstraintForceY=off  SenseConstraintForceZ=off  SenseConstraintTorque=off  SenseConstraintTorqueX=off  SenseConstraintTorqueY=off  SenseConstraintTorqueZ=off  SenseTotalForce=off  SenseTotalForceX=off  SenseTotalForceY=off  SenseTotalForceZ=off  SenseTotalTorque=off  SenseTotalTorqueX=off  SenseTotalTorqueY=off  SenseTotalTorqueZ=off  CompositeWrenchDir=FollowerOnBase  CompositeWrenchFrame=BaseFrame
  joint5_x1_Link : Subsystem
  Conn5 : PMIOPort  Side=Left
  Conn6 : PMIOPort  Port=2  Side=Right
  Out1 : Outport
  wires:
  In1/1 -> Variant Subsystem9/1(In1)
  Variant Subsystem9/1(Out1) -> Out1/1
  connections:
  Conn5/RConn1 -- joint5_Link/LConn1
  Variant Subsystem9/RConn1 -- Conn6/RConn1
  Variant Subsystem9/LConn1 -- joint5_Link/RConn1
  joint5_x1/RConn1 -- joint5_x1_Link/LConn1
  joint5_Link/RConn2 -- joint5_x1/LConn1

== system PID_Joint23_Simscape_Simulation/Subsystem2/joint6_Link ==
  Inertia : sm_lib/Body Elements/Inertia  InertiaType=Custom  Mass=0.065416  MassUnits=kg  CenterOfMass=[0, 0, 0]  CenterOfMassUnits=m  MomentsOfInertia=[3.1992e-05, 3.1414e-05, 5.9343e-05]  MomentsOfInertiaUnits=kg*m^2  ProductsOfInertia=[-9.5152e-08, -2.0078e-11, -1.1746e-09]  ProductsOfInertiaUnits=kg*m^2  GraphicType=None  MarkerShape=Inertia  MarkerSize=20  GraphicVisPropType=SimpleVisualProperties  GraphicDiffuseColor=[0.5 0.5 0.5]  GraphicSpecularColor=[0.5 0.5 0.5 1.0]  GraphicAmbientColor=[0.15 0.15 0.15 1.0]  GraphicEmissiveColor=[0.0 0.0 0.0 1.0]  GraphicShininess=75  GraphicOpacity=1.0
  InertiaOriginTransform : sm_lib/Frames and Transforms/Rigid Transform  TranslationMethod=Cartesian  TranslationStandardOffset=0  TranslationLengthUnit=m  TranslationStandardAxis=+Z  TranslationCartesianOffset=[9.6535e-05, 0.00028572, -0.016515]  TranslationROffset=0  TranslationROffsetUnits=m  TranslationZOffset=0  TranslationZOffsetUnits=m  TranslationThetaOffset=0  TranslationThetaOffsetUnits=deg  RotationMethod=RotationSequence  RotationAngleUnits=deg  RotationStandardAxis=+Z  RotationAngle=0.0  RotationArbitraryAxis=[0 0 1]  FollAlignAxisA=+X  BaseAlignAxisA=+Y  FollAlignAxisB=+Y  BaseAlignAxisB=+Z  RotationSequenceAxes=BaseAxes  RotationSequence=XYZ  RotationSequenceAngles=[0, 0, 0]  RotationSequenceAnglesUnits=rad  RotationMatrix=[1 0 0; 0 1 0; 0 0 1]
  ReferenceFrame : sm_lib/Frames and Transforms/Reference Frame
  Visual : sm_lib/Body Elements/File Solid  ExtGeomFileName=vscr6/meshes/joint6_Link.STL  UnitType=Custom  ExtGeomFileUnits=m  StepReaderType=HEX  ExportConvexHullGeometry=off  InertiaType=Custom  Mass=0  MassUnits=kg  CenterOfMass=[0, 0, 0]  CenterOfMassUnits=m  MomentsOfInertia=[0, 0, 0]  MomentsOfInertiaUnits=kg*m^2  ProductsOfInertia=[0, 0, 0]  ProductsOfInertiaUnits=kg*m^2  BasedOnType=DensityFromFile  Density=1000  DensityUnits=kg/m^3  DoExposeReferenceFrame=on  SerializedFrames=<Frames/>  GraphicType=FromGeometry  MarkerShape=Sphere  MarkerSize=10  GraphicVisPropType=SimpleVisualProperties  GraphicDiffuseColor=[0.79216, 0.8196099999999999, 0.93333]  GraphicSpecularColor=[0.5 0.5 0.5 1.0]  GraphicAmbientColor=[0.15 0.15 0.15 1.0]  GraphicEmissiveColor=[0.0 0.0 0.0 1.0]  GraphicShininess=75  GraphicOpacity=1
  VisualOriginTransform : sm_lib/Frames and Transforms/Rigid Transform  TranslationMethod=Cartesian  TranslationStandardOffset=0  TranslationLengthUnit=m  TranslationStandardAxis=+Z  TranslationCartesianOffset=[0, 0, 0]  TranslationROffset=0  TranslationROffsetUnits=m  TranslationZOffset=0  TranslationZOffsetUnits=m  TranslationThetaOffset=0  TranslationThetaOffsetUnits=deg  RotationMethod=RotationSequence  RotationAngleUnits=deg  RotationStandardAxis=+Z  RotationAngle=0.0  RotationArbitraryAxis=[0 0 1]  FollAlignAxisA=+X  BaseAlignAxisA=+Y  FollAlignAxisB=+Y  BaseAlignAxisB=+Z  RotationSequenceAxes=BaseAxes  RotationSequence=XYZ  RotationSequenceAngles=[0, 0, 0]  RotationSequenceAnglesUnits=rad  RotationMatrix=[1 0 0; 0 1 0; 0 0 1]
  joint6_AxisInvTransform : sm_lib/Frames and Transforms/Rigid Transform  TranslationMethod=Cartesian  TranslationStandardOffset=0  TranslationLengthUnit=m  TranslationStandardAxis=+Z  TranslationCartesianOffset=[0, 0, 0]  TranslationROffset=0  TranslationROffsetUnits=m  TranslationZOffset=0  TranslationZOffsetUnits=m  TranslationThetaOffset=0  TranslationThetaOffsetUnits=deg  RotationMethod=ArbitraryAxis  RotationAngleUnits=rad  RotationStandardAxis=+Z  RotationAngle=3.141592653589793  RotationArbitraryAxis=[1, 0, 0]  FollAlignAxisA=+X  BaseAlignAxisA=+Y  FollAlignAxisB=+Y  BaseAlignAxisB=+Z  RotationSequenceAxes=FollowerAxes  RotationSequence=XYX  RotationSequenceAngles=[0 0 0]  RotationSequenceAnglesUnits=deg  RotationMatrix=[1 0 0; 0 1 0; 0 0 1]
  F : PMIOPort  Side=Left
  connections:
  Inertia/RConn1 -- InertiaOriginTransform/RConn1
  ReferenceFrame/RConn1 -- InertiaOriginTransform/LConn1 -- VisualOriginTransform/LConn1 -- joint6_AxisInvTransform/LConn1
  Visual/RConn1 -- VisualOriginTransform/RConn1
  joint6_AxisInvTransform/RConn1 -- F/RConn1

== system PID_Joint23_Simscape_Simulation/PIDController/Error2/Subsystem ==
  note: $e_1(t)=\theta(t)-\theta_d(t)$
  position : Inport
  Amplitude : Inport  Port=2
  Enable : EnablePort
  Product : Product
  Sum5 : Sum  Inputs=-+|
  ref_signal : dspsrcs4/Sine Wave  Amplitude=1  Frequency=1/4  Phase=0  SampleMode=Discrete  OutComplex=Real  CompMethod=Trigonometric fcn  TableSize=Speed  SampleTime=0.001  SamplesPerFrame=1  ResetState=Restart at time zero  OutputFrames=on  dataType=double  wordLen=16  udDataType=sfix(16)  fracBitsMode=Best precision  numFracBits=15  OutDataTypeStr=double  LastOutDataTypeStr=double
  限幅 : Saturate  UpperLimit=pi/3  LowerLimit=0
  e1 : Outport  VectorParamsAs1DForOutWhenUnconnected=off
  理想位置 : Outport  Port=2  VectorParamsAs1DForOutWhenUnconnected=off
  wires:
  ref_signal/1 -> Product/1
  position/1 -> Sum5/1
  Sum5/1 -> e1/1
  Product/1 -> Sum5/2, 理想位置/1
  Amplitude/1 -> 限幅/1
  限幅/1 -> Product/2

== system PID_Joint23_Simscape_Simulation/PIDController/Error3/Subsystem ==
  note: $e_1(t)=\theta(t)-\theta_d(t)$
  position : Inport
  Amplitude : Inport  Port=2
  Enable : EnablePort
  Product : Product
  Sum5 : Sum  Inputs=-+|
  ref_signal : dspsrcs4/Sine Wave  Amplitude=1  Frequency=1/4  Phase=0  SampleMode=Discrete  OutComplex=Real  CompMethod=Trigonometric fcn  TableSize=Speed  SampleTime=0.001  SamplesPerFrame=1  ResetState=Restart at time zero  OutputFrames=on  dataType=double  wordLen=16  udDataType=sfix(16)  fracBitsMode=Best precision  numFracBits=15  OutDataTypeStr=double  LastOutDataTypeStr=double
  限幅 : Saturate  UpperLimit=pi/3  LowerLimit=0
  e1 : Outport  VectorParamsAs1DForOutWhenUnconnected=off
  理想位置 : Outport  Port=2  VectorParamsAs1DForOutWhenUnconnected=off
  wires:
  ref_signal/1 -> Product/1
  position/1 -> Sum5/1
  Sum5/1 -> e1/1
  Product/1 -> Sum5/2, 理想位置/1
  Amplitude/1 -> 限幅/1
  限幅/1 -> Product/2

== system PID_Joint23_Simscape_Simulation/Subsystem2/Joint1/Variant Subsystem3 ==
  note: 1) Add Subsystem or Model blocks as valid variant choices.
      | 2) You cannot connect blocks at this level. At simulation, connectivity is automatically
      | determined, based on the active variant and port name matching.
  In1 : Inport
  PositionControl : Subsystem  VariantControl=PositionControl
  TorqueControl : Subsystem  VariantControl=TorqueControl
  Base : PMIOPort  Side=Left
  follower : PMIOPort  Port=2  Side=Right
  Out1 : Outport

== system PID_Joint23_Simscape_Simulation/Subsystem2/Joint1/base_link ==
  base_link : Subsystem
  F2 : PMIOPort  Side=Right
  F : PMIOPort  Port=2  Side=Left
  connections:
  F2/RConn1 -- base_link/RConn1
  base_link/LConn1 -- F/RConn1

== system PID_Joint23_Simscape_Simulation/Subsystem2/Joint2/Variant Subsystem4 ==
  note: 1) Add Subsystem or Model blocks as valid variant choices.
      | 2) You cannot connect blocks at this level. At simulation, connectivity is automatically
      | determined, based on the active variant and port name matching.
  In1 : Inport
  PositionControl : Subsystem  VariantControl=PositionControl
  TorqueControl : Subsystem  VariantControl=TorqueControl
  Base : PMIOPort  Side=Left
  follower : PMIOPort  Port=2  Side=Right
  Out1 : Outport

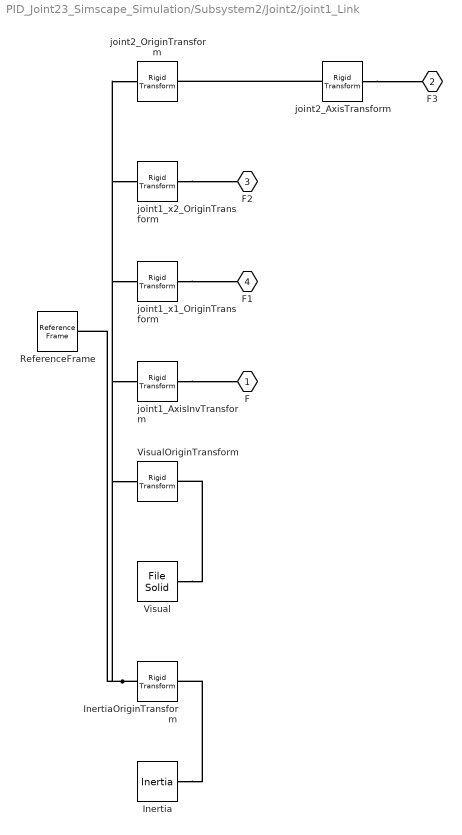
== system PID_Joint23_Simscape_Simulation/Subsystem2/Joint2/joint1_Link ==
  Inertia : sm_lib/Body Elements/Inertia  InertiaType=Custom  Mass=0.80997  MassUnits=kg  CenterOfMass=[0, 0, 0]  CenterOfMassUnits=m  MomentsOfInertia=[0.0012573, 0.0010572, 0.0011455]  MomentsOfInertiaUnits=kg*m^2  ProductsOfInertia=[0.00013038, 4.5862e-09, -3.7432e-09]  ProductsOfInertiaUnits=kg*m^2  GraphicType=None  MarkerShape=Inertia  MarkerSize=20  GraphicVisPropType=SimpleVisualProperties  GraphicDiffuseColor=[0.5 0.5 0.5]  GraphicSpecularColor=[0.5 0.5 0.5 1.0]  GraphicAmbientColor=[0.15 0.15 0.15 1.0]  GraphicEmissiveColor=[0.0 0.0 0.0 1.0]  GraphicShininess=75  GraphicOpacity=1.0
  InertiaOriginTransform : sm_lib/Frames and Transforms/Rigid Transform  TranslationMethod=Cartesian  TranslationStandardOffset=0  TranslationLengthUnit=m  TranslationStandardAxis=+Z  TranslationCartesianOffset=[-5.2679e-07, -0.011954, -0.009115399999999999]  TranslationROffset=0  TranslationROffsetUnits=m  TranslationZOffset=0  TranslationZOffsetUnits=m  TranslationThetaOffset=0  TranslationThetaOffsetUnits=deg  RotationMethod=RotationSequence  RotationAngleUnits=deg  RotationStandardAxis=+Z  RotationAngle=0.0  RotationArbitraryAxis=[0 0 1]  FollAlignAxisA=+X  BaseAlignAxisA=+Y  FollAlignAxisB=+Y  BaseAlignAxisB=+Z  RotationSequenceAxes=BaseAxes  RotationSequence=XYZ  RotationSequenceAngles=[0, 0, 0]  RotationSequenceAnglesUnits=rad  RotationMatrix=[1 0 0; 0 1 0; 0 0 1]
  ReferenceFrame : sm_lib/Frames and Transforms/Reference Frame
  Visual : sm_lib/Body Elements/File Solid  ExtGeomFileName=vscr6/meshes/joint1_Link.STL  UnitType=Custom  ExtGeomFileUnits=m  StepReaderType=HEX  ExportConvexHullGeometry=off  InertiaType=Custom  Mass=0  MassUnits=kg  CenterOfMass=[0, 0, 0]  CenterOfMassUnits=m  MomentsOfInertia=[0, 0, 0]  MomentsOfInertiaUnits=kg*m^2  ProductsOfInertia=[0, 0, 0]  ProductsOfInertiaUnits=kg*m^2  BasedOnType=DensityFromFile  Density=1000  DensityUnits=kg/m^3  DoExposeReferenceFrame=on  SerializedFrames=<Frames/>  GraphicType=FromGeometry  MarkerShape=Sphere  MarkerSize=10  GraphicVisPropType=SimpleVisualProperties  GraphicDiffuseColor=[0.79216, 0.8196099999999999, 0.93333]  GraphicSpecularColor=[0.5 0.5 0.5 1.0]  GraphicAmbientColor=[0.15 0.15 0.15 1.0]  GraphicEmissiveColor=[0.0 0.0 0.0 1.0]  GraphicShininess=75  GraphicOpacity=1
  VisualOriginTransform : sm_lib/Frames and Transforms/Rigid Transform  TranslationMethod=Cartesian  TranslationStandardOffset=0  TranslationLengthUnit=m  TranslationStandardAxis=+Z  TranslationCartesianOffset=[0, 0, 0]  TranslationROffset=0  TranslationROffsetUnits=m  TranslationZOffset=0  TranslationZOffsetUnits=m  TranslationThetaOffset=0  TranslationThetaOffsetUnits=deg  RotationMethod=RotationSequence  RotationAngleUnits=deg  RotationStandardAxis=+Z  RotationAngle=0.0  RotationArbitraryAxis=[0 0 1]  FollAlignAxisA=+X  BaseAlignAxisA=+Y  FollAlignAxisB=+Y  BaseAlignAxisB=+Z  RotationSequenceAxes=BaseAxes  RotationSequence=XYZ  RotationSequenceAngles=[0, 0, 0]  RotationSequenceAnglesUnits=rad  RotationMatrix=[1 0 0; 0 1 0; 0 0 1]
  joint1_AxisInvTransform : sm_lib/Frames and Transforms/Rigid Transform  TranslationMethod=Cartesian  TranslationStandardOffset=0  TranslationLengthUnit=m  TranslationStandardAxis=+Z  TranslationCartesianOffset=[0, 0, 0]  TranslationROffset=0  TranslationROffsetUnits=m  TranslationZOffset=0  TranslationZOffsetUnits=m  TranslationThetaOffset=0  TranslationThetaOffsetUnits=deg  RotationMethod=ArbitraryAxis  RotationAngleUnits=rad  RotationStandardAxis=+Z  RotationAngle=3.141592653589793  RotationArbitraryAxis=[1, 0, 0]  FollAlignAxisA=+X  BaseAlignAxisA=+Y  FollAlignAxisB=+Y  BaseAlignAxisB=+Z  RotationSequenceAxes=FollowerAxes  RotationSequence=XYX  RotationSequenceAngles=[0 0 0]  RotationSequenceAnglesUnits=deg  RotationMatrix=[1 0 0; 0 1 0; 0 0 1]
  joint1_x1_OriginTransform : sm_lib/Frames and Transforms/Rigid Transform  TranslationMethod=Cartesian  TranslationStandardOffset=0  TranslationLengthUnit=m  TranslationStandardAxis=+Z  TranslationCartesianOffset=[0, 0, 0]  TranslationROffset=0  TranslationROffsetUnits=m  TranslationZOffset=0  TranslationZOffsetUnits=m  TranslationThetaOffset=0  TranslationThetaOffsetUnits=deg  RotationMethod=RotationSequence  RotationAngleUnits=deg  RotationStandardAxis=+Z  RotationAngle=0.0  RotationArbitraryAxis=[0 0 1]  FollAlignAxisA=+X  BaseAlignAxisA=+Y  FollAlignAxisB=+Y  BaseAlignAxisB=+Z  RotationSequenceAxes=BaseAxes  RotationSequence=XYZ  RotationSequenceAngles=[0, 0, 0]  RotationSequenceAnglesUnits=rad  RotationMatrix=[1 0 0; 0 1 0; 0 0 1]
  joint1_x2_OriginTransform : sm_lib/Frames and Transforms/Rigid Transform  TranslationMethod=Cartesian  TranslationStandardOffset=0  TranslationLengthUnit=m  TranslationStandardAxis=+Z  TranslationCartesianOffset=[0, 0, 0]  TranslationROffset=0  TranslationROffsetUnits=m  TranslationZOffset=0  TranslationZOffsetUnits=m  TranslationThetaOffset=0  TranslationThetaOffsetUnits=deg  RotationMethod=RotationSequence  RotationAngleUnits=deg  RotationStandardAxis=+Z  RotationAngle=0.0  RotationArbitraryAxis=[0 0 1]  FollAlignAxisA=+X  BaseAlignAxisA=+Y  FollAlignAxisB=+Y  BaseAlignAxisB=+Z  RotationSequenceAxes=BaseAxes  RotationSequence=XYZ  RotationSequenceAngles=[0, 0, 0]  RotationSequenceAnglesUnits=rad  RotationMatrix=[1 0 0; 0 1 0; 0 0 1]
  joint2_AxisTransform : sm_lib/Frames and Transforms/Rigid Transform  TranslationMethod=Cartesian  TranslationStandardOffset=0  TranslationLengthUnit=m  TranslationStandardAxis=+Z  TranslationCartesianOffset=[0, 0, 0]  TranslationROffset=0  TranslationROffsetUnits=m  TranslationZOffset=0  TranslationZOffsetUnits=m  TranslationThetaOffset=0  TranslationThetaOffsetUnits=deg  RotationMethod=ArbitraryAxis  RotationAngleUnits=rad  RotationStandardAxis=+Z  RotationAngle=1.570796326794897  RotationArbitraryAxis=[-1, 0, 0]  FollAlignAxisA=+X  BaseAlignAxisA=+Y  FollAlignAxisB=+Y  BaseAlignAxisB=+Z  RotationSequenceAxes=FollowerAxes  RotationSequence=XYX  RotationSequenceAngles=[0 0 0]  RotationSequenceAnglesUnits=deg  RotationMatrix=[1 0 0; 0 1 0; 0 0 1]
  joint2_OriginTransform : sm_lib/Frames and Transforms/Rigid Transform  TranslationMethod=Cartesian  TranslationStandardOffset=0  TranslationLengthUnit=m  TranslationStandardAxis=+Z  TranslationCartesianOffset=[0, -0.1271, 0]  TranslationROffset=0  TranslationROffsetUnits=m  TranslationZOffset=0  TranslationZOffsetUnits=m  TranslationThetaOffset=0  TranslationThetaOffsetUnits=deg  RotationMethod=RotationSequence  RotationAngleUnits=deg  RotationStandardAxis=+Z  RotationAngle=0.0  RotationArbitraryAxis=[0 0 1]  FollAlignAxisA=+X  BaseAlignAxisA=+Y  FollAlignAxisB=+Y  BaseAlignAxisB=+Z  RotationSequenceAxes=BaseAxes  RotationSequence=XYZ  RotationSequenceAngles=[0, 0, 0]  RotationSequenceAnglesUnits=rad  RotationMatrix=[1 0 0; 0 1 0; 0 0 1]
  F : PMIOPort  Side=Left
  F3 : PMIOPort  Port=2  Side=Right
  F2 : PMIOPort  Port=3  Side=Right
  F1 : PMIOPort  Port=4  Side=Right
  connections:
  Inertia/RConn1 -- InertiaOriginTransform/RConn1
  ReferenceFrame/RConn1 -- InertiaOriginTransform/LConn1 -- VisualOriginTransform/LConn1 -- joint1_AxisInvTransform/LConn1 -- joint1_x1_OriginTransform/LConn1 -- joint1_x2_OriginTransform/LConn1 -- joint2_OriginTransform/LConn1
  Visual/RConn1 -- VisualOriginTransform/RConn1
  joint1_AxisInvTransform/RConn1 -- F/RConn1
  joint1_x1_OriginTransform/RConn1 -- F1/RConn1
  joint1_x2_OriginTransform/RConn1 -- F2/RConn1
  joint2_AxisTransform/RConn1 -- F3/RConn1
  joint2_AxisTransform/LConn1 -- joint2_OriginTransform/RConn1

== system PID_Joint23_Simscape_Simulation/Subsystem2/Joint2/joint1_x1_Link ==
  Inertia : sm_lib/Body Elements/Inertia  InertiaType=Custom  Mass=0.24441  MassUnits=kg  CenterOfMass=[0, 0, 0]  CenterOfMassUnits=m  MomentsOfInertia=[0.0001565, 0.00016175, 0.00024408]  MomentsOfInertiaUnits=kg*m^2  ProductsOfInertia=[2.2617e-05, 1.8263e-07, -1.2509e-07]  ProductsOfInertiaUnits=kg*m^2  GraphicType=None  MarkerShape=Inertia  MarkerSize=20  GraphicVisPropType=SimpleVisualProperties  GraphicDiffuseColor=[0.5 0.5 0.5]  GraphicSpecularColor=[0.5 0.5 0.5 1.0]  GraphicAmbientColor=[0.15 0.15 0.15 1.0]  GraphicEmissiveColor=[0.0 0.0 0.0 1.0]  GraphicShininess=75  GraphicOpacity=1.0
  InertiaOriginTransform : sm_lib/Frames and Transforms/Rigid Transform  TranslationMethod=Cartesian  TranslationStandardOffset=0  TranslationLengthUnit=m  TranslationStandardAxis=+Z  TranslationCartesianOffset=[-5.654e-05, 0.0055654, 0.051426]  TranslationROffset=0  TranslationROffsetUnits=m  TranslationZOffset=0  TranslationZOffsetUnits=m  TranslationThetaOffset=0  TranslationThetaOffsetUnits=deg  RotationMethod=RotationSequence  RotationAngleUnits=deg  RotationStandardAxis=+Z  RotationAngle=0.0  RotationArbitraryAxis=[0 0 1]  FollAlignAxisA=+X  BaseAlignAxisA=+Y  FollAlignAxisB=+Y  BaseAlignAxisB=+Z  RotationSequenceAxes=BaseAxes  RotationSequence=XYZ  RotationSequenceAngles=[0, 0, 0]  RotationSequenceAnglesUnits=rad  RotationMatrix=[1 0 0; 0 1 0; 0 0 1]
  ReferenceFrame : sm_lib/Frames and Transforms/Reference Frame
  Visual : sm_lib/Body Elements/File Solid  ExtGeomFileName=vscr6/meshes/joint1_x1_Link.STL  UnitType=Custom  ExtGeomFileUnits=m  StepReaderType=HEX  ExportConvexHullGeometry=off  InertiaType=Custom  Mass=0  MassUnits=kg  CenterOfMass=[0, 0, 0]  CenterOfMassUnits=m  MomentsOfInertia=[0, 0, 0]  MomentsOfInertiaUnits=kg*m^2  ProductsOfInertia=[0, 0, 0]  ProductsOfInertiaUnits=kg*m^2  BasedOnType=DensityFromFile  Density=1000  DensityUnits=kg/m^3  DoExposeReferenceFrame=on  SerializedFrames=<Frames/>  GraphicType=FromGeometry  MarkerShape=Sphere  MarkerSize=10  GraphicVisPropType=SimpleVisualProperties  GraphicDiffuseColor=[0, 0.5, 0]  GraphicSpecularColor=[0.5 0.5 0.5 1.0]  GraphicAmbientColor=[0.15 0.15 0.15 1.0]  GraphicEmissiveColor=[0.0 0.0 0.0 1.0]  GraphicShininess=75  GraphicOpacity=1
  VisualOriginTransform : sm_lib/Frames and Transforms/Rigid Transform  TranslationMethod=Cartesian  TranslationStandardOffset=0  TranslationLengthUnit=m  TranslationStandardAxis=+Z  TranslationCartesianOffset=[0, 0, 0]  TranslationROffset=0  TranslationROffsetUnits=m  TranslationZOffset=0  TranslationZOffsetUnits=m  TranslationThetaOffset=0  TranslationThetaOffsetUnits=deg  RotationMethod=RotationSequence  RotationAngleUnits=deg  RotationStandardAxis=+Z  RotationAngle=0.0  RotationArbitraryAxis=[0 0 1]  FollAlignAxisA=+X  BaseAlignAxisA=+Y  FollAlignAxisB=+Y  BaseAlignAxisB=+Z  RotationSequenceAxes=BaseAxes  RotationSequence=XYZ  RotationSequenceAngles=[0, 0, 0]  RotationSequenceAnglesUnits=rad  RotationMatrix=[1 0 0; 0 1 0; 0 0 1]
  F : PMIOPort  Side=Left
  connections:
  Inertia/RConn1 -- InertiaOriginTransform/RConn1
  ReferenceFrame/RConn1 -- InertiaOriginTransform/LConn1 -- VisualOriginTransform/LConn1 -- F/RConn1
  Visual/RConn1 -- VisualOriginTransform/RConn1
